simulink model "DecentralizedLFADRC"  (R2019b)
settings: Solver=ode4  StartTime=0.0  StopTime=480  FixedStep=1e-3  MaxStep=1e-4  RelTol=1e-3  EnableMultiTasking=on
values from neighbouring files (symbols this model uses):
  a_1 = 0.5    [system_parameters.m]
  a_10 = 0.125    [system_parameters.m]
  a_2 = 0.125    [system_parameters.m]
  a_3 = 0.125    [system_parameters.m]
  a_4 = 0.5    [system_parameters.m]
  a_5 = 0.1    [system_parameters.m]
  a_6 = 0.1    [system_parameters.m]
  a_7 = 0.1    [system_parameters.m]
  a_8 = 0.125    [system_parameters.m]
  a_9 = 0.5    [system_parameters.m]
  a_PV1 = 0.125    [system_parameters.m]
  a_PV2 = 0.2    [system_parameters.m]
  a_PV3 = 0.125    [system_parameters.m]
  a_WT1 = 0.125    [system_parameters.m]
  a_WT3 = 0.125    [system_parameters.m]
  B1 = (1/Req1)+D    [system_parameters.m]
  B2 = (1/Req2)+D    [system_parameters.m]
  B3 = (1/Req3)+D    [system_parameters.m]
  D = 2    [system_parameters.m]
  H_A1 = (H1*S1+H2*S2+H3*S3)/(S1+S2+S3)    (= 2.58715528865)    [system_parameters.m]
  H_A2 = (H4*S4+H5*S5+H6*S6+H7*S7)/(S4+S5+S6+S7)    (= 2.6419)    [system_parameters.m]
  H_A3 = (H8*S8+H9*S9+H10*S10)/(S8+S9+S10)    (= 2.49952427226)    [system_parameters.m]
  K1 = -K1    [design_LFADRC.m]
  K2 = -K2    [design_LFADRC.m]
  K3 = -K3    [design_LFADRC.m]
  kpc = 0.8    [system_parameters.m]
  R1 = 0.0548    [system_parameters.m]
  R4 = 0.06    [system_parameters.m]
  R9 = 0.0548    [system_parameters.m]
  Rp10 = 0.06    [system_parameters.m]
  Rp2 = 0.06    [system_parameters.m]
  Rp3 = 0.06    [system_parameters.m]
  Rp5 = 0.0548    [system_parameters.m]
  Rp6 = 0.06    [system_parameters.m]
  Rp7 = 0.06    [system_parameters.m]
  Rp8 = 0.06    [system_parameters.m]
  RPV1 = 0.05    [system_parameters.m]
  RPV2 = 0.05    [system_parameters.m]
  RPV3 = 0.05    [system_parameters.m]
  RWT1 = 0.024    [system_parameters.m]
  RWT3 = 0.024    [system_parameters.m]
  T12 = 2.5    [system_parameters.m]
  T13 = 5.0    (= 5)    [system_parameters.m]
  T23 = 3.8    [system_parameters.m]
undefined symbols (not defined in the file or in its folder): A_obs_1, A_obs_2, A_obs_3, B_obs_1, B_obs_2, B_obs_3, C_obs_1, C_obs_2, C_obs_3, D_obs_1, D_obs_2, D_obs_3, X_hat_1, X_hat_2, X_hat_3, Xi_hat_1, Xi_hat_2, Xi_hat_3
libraries: cstblocks x94, simulink x40
(part 1 of 2)
settings Model: Creator=sergi  LastModifiedBy=sergio.dorado
settings DataIOCC: LimitDataPoints=on  SaveFormat=Array  ReturnWorkspaceOutputs=off
settings OptimizationCC: LifeSpan=inf
settings DebuggingCC: SFUnexpectedBacktrackingDiag=warning  SFNoUnconditionalDefaultTransitionDiag=warning  SFExecutionAtInitializationDiag=none  ArithmeticOperatorsInVariantConditions=warning
settings HardwareCC: ProdBitPerPointer=32  ProdBitPerSizeT=32  ProdBitPerPtrDiffT=32  ProdLargestAtomicFloat=None  ProdIntDivRoundTo=Undefined  ProdEndianess=Unspecified  ProdWordSize=32  ProdHWDeviceType=32-bit Generic
settings ModelReferenceCC: PropagateSignalLabelsOutOfModel=off
settings SFSimCC: SimUseLocalCustomCode=off  CustomCodeUndefinedFunction=UseInterfaceOnly
settings RTWCC: RTWUseLocalCustomCode=off
settings CodeAppCC: StateflowObjectComments=on
settings GRTTargetCC: TargetLangStandard=C89/C90 (ANSI)  GeneratePreprocessorConditionals=Disable all
settings ConfigComp: CovMetricSettings=dw  CovHtmlReporting=on  CovSaveCumulativeToWorkspaceVar=on  CovSaveSingleToWorkspaceVar=on  CovExternalEMLEnable=off

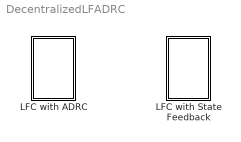
== system DecentralizedLFADRC ==
  LFC with State Feedback : Subsystem
  LFC with ADRC : Subsystem

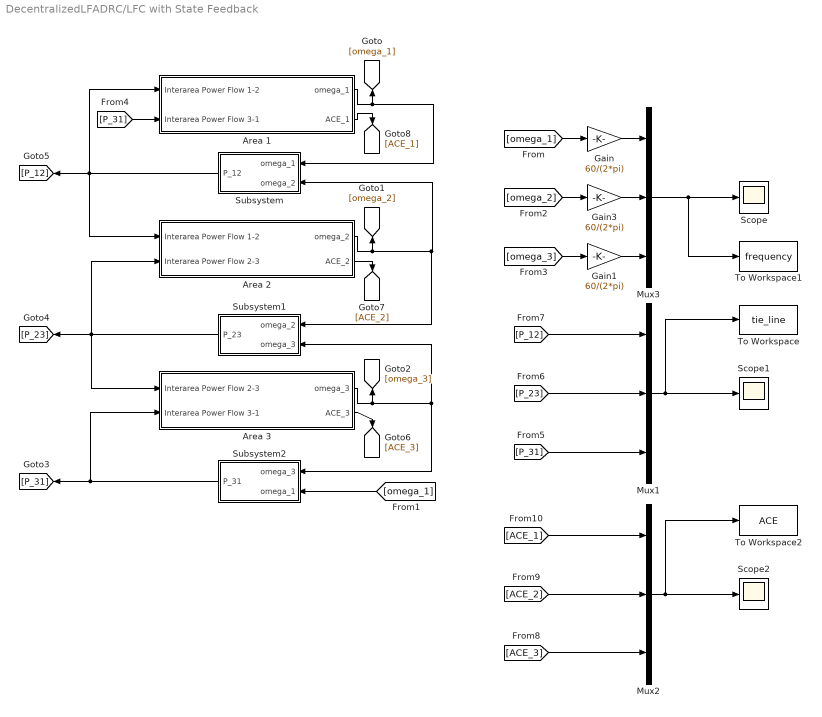
== system DecentralizedLFADRC/LFC with State Feedback ==
  Area 1 : Subsystem
  Area 2 : Subsystem
  Area 3 : Subsystem
  Gain : Gain  Gain=60/(2*pi)
  Gain1 : Gain  Gain=60/(2*pi)
  Gain3 : Gain  Gain=60/(2*pi)
  Mux1 : Mux  Inputs=3
  Mux2 : Mux  Inputs=3
  Mux3 : Mux  Inputs=3
  Scope : Scope
  Scope1 : Scope
  Scope2 : Scope
  Subsystem : Subsystem
  Subsystem1 : Subsystem
  Subsystem2 : Subsystem
  To Workspace : ToWorkspace  VariableName=tie_line  SaveFormat=Structure With Time  SampleTime=-1
  To Workspace1 : ToWorkspace  VariableName=frequency  SaveFormat=Structure With Time  SampleTime=-1
  To Workspace2 : ToWorkspace  VariableName=ACE  SaveFormat=Structure With Time  SampleTime=-1
  wires:
  Gain3/1 -> Mux3/2
  Area 3/1(omega_3) -> Subsystem2/1(omega_3), Subsystem1/2(omega_3), [omega_3]
  Mux3/1 -> To Workspace1/1, Scope/1
  [P_12] -> Mux1/1
  Mux1/1 -> To Workspace/1, Scope1/1
  [omega_1] -> Gain/1
  Area 2/1(omega_2) -> Subsystem1/1(omega_2), Subsystem/2(omega_2), [omega_2]
  Area 1/1(omega_1) -> Subsystem/1(omega_1), [omega_1]
  Gain/1 -> Mux3/1
  [P_31] -> Mux1/3
  Subsystem2/1(P_31) -> [P_31], Area 3/2(Interarea Power Flow 3-1)
  Subsystem/1(P_12) -> [P_12], Area 2/1(Interarea Power Flow 1-2), Area 1/1(Interarea Power Flow 1-2)
  [omega_2] -> Gain3/1
  [omega_1] -> Subsystem2/2(omega_1)
  [P_31] -> Area 1/2(Interarea Power Flow 3-1)
  [omega_3] -> Gain1/1
  Subsystem1/1(P_23) -> [P_23], Area 3/1(Interarea Power Flow 2-3), Area 2/2(Interarea Power Flow 2-3)
  Gain1/1 -> Mux3/3
  [P_23] -> Mux1/2
  [ACE_1] -> Mux2/1
  [ACE_2] -> Mux2/2
  [ACE_3] -> Mux2/3
  Mux2/1 -> Scope2/1, To Workspace2/1
  Area 3/2(ACE_3) -> [ACE_3]
  Area 2/2(ACE_2) -> [ACE_2]
  Area 1/2(ACE_1) -> [ACE_1]

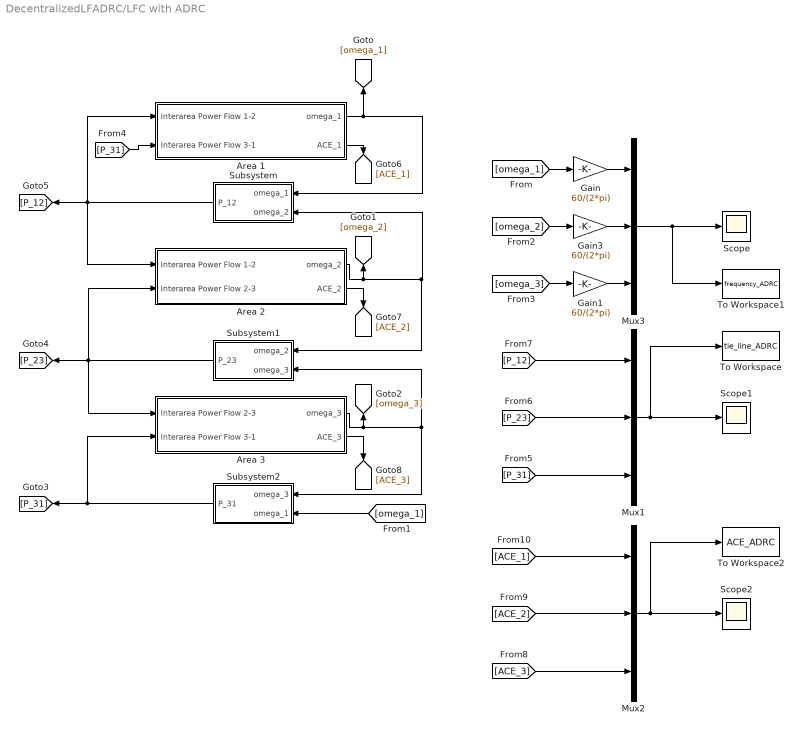
== system DecentralizedLFADRC/LFC with ADRC ==
  Area 1 : Subsystem
  Area 2 : Subsystem
  Area 3 : Subsystem
  Gain : Gain  Gain=60/(2*pi)
  Gain1 : Gain  Gain=60/(2*pi)
  Gain3 : Gain  Gain=60/(2*pi)
  Mux1 : Mux  Inputs=3
  Mux2 : Mux  Inputs=3
  Mux3 : Mux  Inputs=3
  Scope : Scope
  Scope1 : Scope
  Scope2 : Scope
  Subsystem : Subsystem
  Subsystem1 : Subsystem
  Subsystem2 : Subsystem
  To Workspace : ToWorkspace  VariableName=tie_line_ADRC  SaveFormat=Structure With Time  SampleTime=-1
  To Workspace1 : ToWorkspace  VariableName=frequency_ADRC  SaveFormat=Structure With Time  SampleTime=-1
  To Workspace2 : ToWorkspace  VariableName=ACE_ADRC  SaveFormat=Structure With Time  SampleTime=-1
  wires:
  [P_23] -> Mux1/2
  Gain1/1 -> Mux3/3
  Subsystem1/1(P_23) -> Area 2/2(Interarea Power Flow 2-3), Area 3/1(Interarea Power Flow 2-3), [P_23]
  [omega_3] -> Gain1/1
  [P_31] -> Area 1/2(Interarea Power Flow 3-1)
  [omega_1] -> Subsystem2/2(omega_1)
  [omega_2] -> Gain3/1
  Subsystem/1(P_12) -> Area 1/1(Interarea Power Flow 1-2), Area 2/1(Interarea Power Flow 1-2), [P_12]
  Subsystem2/1(P_31) -> Area 3/2(Interarea Power Flow 3-1), [P_31]
  [P_31] -> Mux1/3
  Gain/1 -> Mux3/1
  Area 1/1(omega_1) -> Subsystem/1(omega_1), [omega_1]
  Area 2/1(omega_2) -> [omega_2], Subsystem/2(omega_2), Subsystem1/1(omega_2)
  [omega_1] -> Gain/1
  Mux1/1 -> Scope1/1, To Workspace/1
  [P_12] -> Mux1/1
  Mux3/1 -> Scope/1, To Workspace1/1
  Area 3/1(omega_3) -> [omega_3], Subsystem1/2(omega_3), Subsystem2/1(omega_3)
  Gain3/1 -> Mux3/2
  [ACE_3] -> Mux2/3
  Mux2/1 -> Scope2/1, To Workspace2/1
  [ACE_1] -> Mux2/1
  [ACE_2] -> Mux2/2
  Area 1/2(ACE_1) -> [ACE_1]
  Area 2/2(ACE_2) -> [ACE_2]
  Area 3/2(ACE_3) -> [ACE_3]

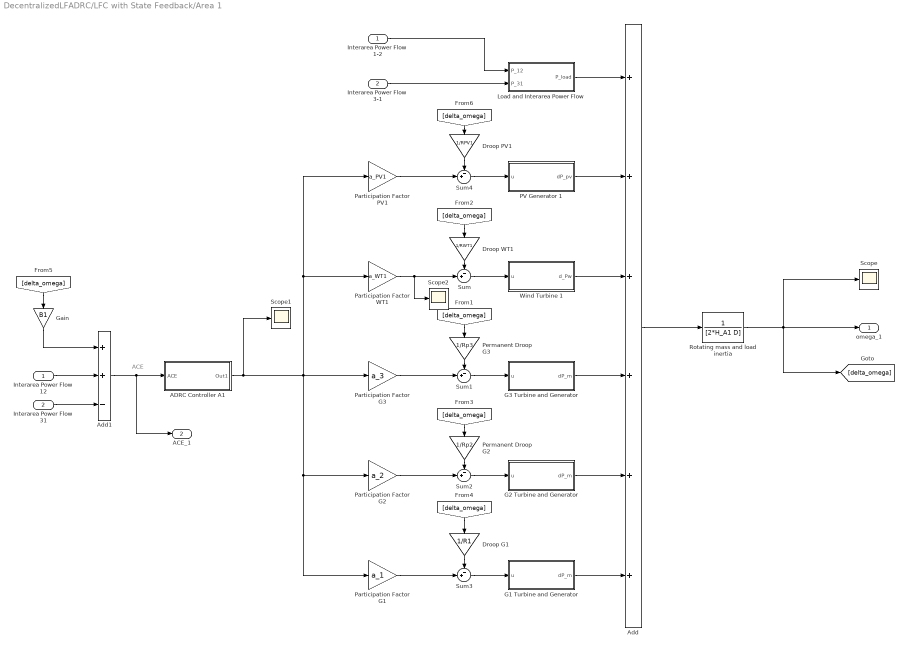
== system DecentralizedLFADRC/LFC with State Feedback/Area 1 ==
  note: ACE
  Interarea Power Flow 1-2 : Inport
  Interarea Power Flow 3-1 : Inport  Port=2
  ADRC Controller A1 : Subsystem
  Add : Sum  Inputs=6
  Add1 : Sum  Inputs=++-
  Droop G1 : Gain  Gain=1/R1
  Droop PV1 : Gain  Gain=1/RPV1
  Droop WT1 : Gain  Gain=1/RWT1
  G1 Turbine and Generator : Subsystem
  G2 Turbine and Generator : Subsystem
  G3 Turbine and Generator : Subsystem
  Gain : Gain  Gain=B1
  Interarea Power Flow 12 : InportShadow
  Interarea Power Flow 31 : InportShadow  Port=2
  Load and Interarea Power Flow : Subsystem
  "PV Generator 1 " : Subsystem
  Participation Factor G1 : Gain  Gain=a_1
  Participation Factor G2 : Gain  Gain=a_2
  Participation Factor G3 : Gain  Gain=a_3
  Participation Factor PV1 : Gain  Gain=a_PV1
  Participation Factor WT1 : Gain  Gain=a_WT1
  Permanent Droop G2 : Gain  Gain=1/Rp2
  Permanent Droop G3 : Gain  Gain=1/Rp3
  Rotating mass and load inertia : TransferFcn  Denominator=[2*H_A1 D]
  Scope : Scope
  Scope1 : Scope
  Scope2 : Scope
  Sum{,1..4} (5 alike) : Sum  Inputs=-+|
  Wind Turbine 1 : Subsystem
  omega_1 : Outport  VectorParamsAs1DForOutWhenUnconnected=off
  ACE_1 : Outport  Port=2  VectorParamsAs1DForOutWhenUnconnected=off
  wires:
  Rotating mass and load inertia/1 -> omega_1/1, Scope/1, [delta_omega]
  Add/1 -> Rotating mass and load inertia/1
  Sum/1 -> Wind Turbine 1/1(u)
  Sum1/1 -> G3 Turbine and Generator/1(u)
  Sum2/1 -> G2 Turbine and Generator/1(u)
  Droop G1/1 -> Sum3/1
  [delta_omega] -> Droop G1/1
  Participation Factor WT1/1 -> Scope2/1, Sum/2
  Participation Factor G3/1 -> Sum1/2
  Participation Factor G2/1 -> Sum2/2
  Participation Factor G1/1 -> Sum3/2
  Permanent Droop G2/1 -> Sum2/1
  [delta_omega] -> Permanent Droop G2/1
  Permanent Droop G3/1 -> Sum1/1
  [delta_omega] -> Permanent Droop G3/1
  Droop WT1/1 -> Sum/1
  [delta_omega] -> Droop WT1/1
  Interarea Power Flow 1-2/1 -> Load and Interarea Power Flow/1(P_12)
  Interarea Power Flow 3-1/1 -> Load and Interarea Power Flow/2(P_31)
  Sum3/1 -> G1 Turbine and Generator/1(u)
  G1 Turbine and Generator/1(dP_m) -> Add/6
  G2 Turbine and Generator/1(dP_m) -> Add/5
  G3 Turbine and Generator/1(dP_m) -> Add/4
  Wind Turbine 1/1(d_Pw) -> Add/3
  [delta_omega] -> Droop PV1/1
  Droop PV1/1 -> Sum4/1
  Participation Factor PV1/1 -> Sum4/2
  Sum4/1 -> "PV Generator 1 "/1(u)
  "PV Generator 1 "/1(dP_pv) -> Add/2
  Load and Interarea Power Flow/1(P_load) -> Add/1
  Add1/1 -> ACE_1/1, ADRC Controller A1/1(ACE)
  [delta_omega] -> Gain/1
  Gain/1 -> Add1/1
  Interarea Power Flow 31/1 -> Add1/3
  Interarea Power Flow 12/1 -> Add1/2
  ADRC Controller A1/1(Out1) -> Participation Factor WT1/1, Participation Factor PV1/1, Participation Factor G3/1, Participation Factor G1/1, Participation Factor G2/1, Scope1/1

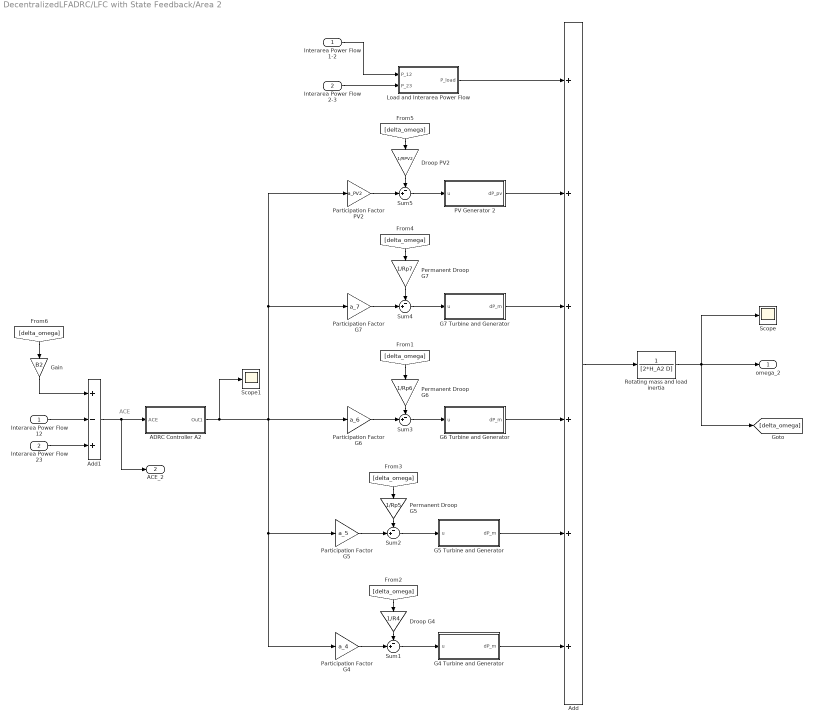
== system DecentralizedLFADRC/LFC with State Feedback/Area 2 ==
  note: ACE
  Interarea Power Flow 1-2 : Inport
  Interarea Power Flow 2-3 : Inport  Port=2
  ADRC Controller A2 : Subsystem
  Add : Sum  Inputs=6
  Add1 : Sum  Inputs=+-+
  Droop G4 : Gain  Gain=1/R4
  Droop PV2 : Gain  Gain=1/RPV2
  G4 Turbine and Generator : Subsystem
  G5 Turbine and Generator : Subsystem
  G6 Turbine and Generator : Subsystem
  G7 Turbine and Generator : Subsystem
  Gain : Gain  Gain=B2
  Interarea Power Flow 12 : InportShadow
  Interarea Power Flow 23 : InportShadow  Port=2
  Load and Interarea Power Flow : Subsystem
  "PV Generator 2 " : Subsystem
  Participation Factor G4 : Gain  Gain=a_4
  Participation Factor G5 : Gain  Gain=a_5
  Participation Factor G6 : Gain  Gain=a_6
  Participation Factor G7 : Gain  Gain=a_7
  Participation Factor PV2 : Gain  Gain=a_PV2
  Permanent Droop G5 : Gain  Gain=1/Rp5
  Permanent Droop G6 : Gain  Gain=1/Rp6
  Permanent Droop G7 : Gain  Gain=1/Rp7
  Rotating mass and load inertia : TransferFcn  Denominator=[2*H_A2 D]
  Scope : Scope
  Scope1 : Scope
  Sum{1..5} (5 alike) : Sum  Inputs=-+|
  omega_2 : Outport  VectorParamsAs1DForOutWhenUnconnected=off
  ACE_2 : Outport  Port=2  VectorParamsAs1DForOutWhenUnconnected=off
  wires:
  Add/1 -> Rotating mass and load inertia/1
  Rotating mass and load inertia/1 -> omega_2/1, Scope/1, [delta_omega]
  Sum4/1 -> G7 Turbine and Generator/1(u)
  Droop G4/1 -> Sum1/1
  [delta_omega] -> Droop G4/1
  Sum1/1 -> G4 Turbine and Generator/1(u)
  Participation Factor G4/1 -> Sum1/2
  Permanent Droop G5/1 -> Sum2/1
  [delta_omega] -> Permanent Droop G5/1
  Participation Factor G5/1 -> Sum2/2
  Sum2/1 -> G5 Turbine and Generator/1(u)
  Sum3/1 -> G6 Turbine and Generator/1(u)
  Permanent Droop G6/1 -> Sum3/1
  Participation Factor G6/1 -> Sum3/2
  [delta_omega] -> Permanent Droop G6/1
  [delta_omega] -> Permanent Droop G7/1
  Permanent Droop G7/1 -> Sum4/1
  Participation Factor G7/1 -> Sum4/2
  Sum5/1 -> "PV Generator 2 "/1(u)
  Participation Factor PV2/1 -> Sum5/2
  [delta_omega] -> Droop PV2/1
  Droop PV2/1 -> Sum5/1
  Load and Interarea Power Flow/1(P_load) -> Add/1
  ADRC Controller A2/1(Out1) -> Scope1/1, Participation Factor G4/1, Participation Factor G5/1, Participation Factor G6/1, Participation Factor PV2/1, Participation Factor G7/1
  Interarea Power Flow 2-3/1 -> Load and Interarea Power Flow/2(P_23)
  Interarea Power Flow 1-2/1 -> Load and Interarea Power Flow/1(P_12)
  G4 Turbine and Generator/1(dP_m) -> Add/6
  "PV Generator 2 "/1(dP_pv) -> Add/2
  Interarea Power Flow 23/1 -> Add1/3
  Gain/1 -> Add1/1
  Add1/1 -> ACE_2/1, ADRC Controller A2/1(ACE)
  Interarea Power Flow 12/1 -> Add1/2
  [delta_omega] -> Gain/1
  G7 Turbine and Generator/1(dP_m) -> Add/3
  G6 Turbine and Generator/1(dP_m) -> Add/4
  G5 Turbine and Generator/1(dP_m) -> Add/5

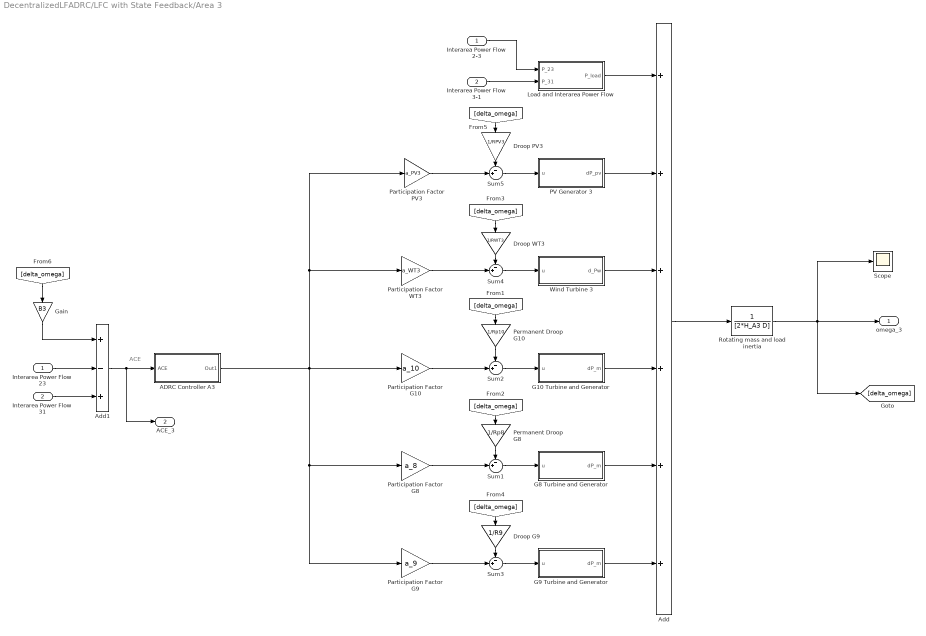
== system DecentralizedLFADRC/LFC with State Feedback/Area 3 ==
  note: ACE
  Interarea Power Flow 2-3 : Inport
  Interarea Power Flow 3-1 : Inport  Port=2
  ADRC Controller A3 : Subsystem
  Add : Sum  Inputs=6
  Add1 : Sum  Inputs=+-+
  Droop G9 : Gain  Gain=1/R9
  Droop PV3 : Gain  Gain=1/RPV3
  Droop WT3 : Gain  Gain=1/RWT3
  G10 Turbine and Generator : Subsystem
  G8 Turbine and Generator : Subsystem
  G9 Turbine and Generator : Subsystem
  Gain : Gain  Gain=B3
  Interarea Power Flow 23 : InportShadow
  Interarea Power Flow 31 : InportShadow  Port=2
  Load and Interarea Power Flow : Subsystem
  "PV Generator 3 " : Subsystem
  Participation Factor G10 : Gain  Gain=a_10
  Participation Factor G8 : Gain  Gain=a_8
  Participation Factor G9 : Gain  Gain=a_9
  Participation Factor PV3 : Gain  Gain=a_PV3
  Participation Factor WT3 : Gain  Gain=a_WT3
  Permanent Droop G10 : Gain  Gain=1/Rp10
  Permanent Droop G8 : Gain  Gain=1/Rp8
  Rotating mass and load inertia : TransferFcn  Denominator=[2*H_A3 D]
  Scope : Scope
  Sum{1..5} (5 alike) : Sum  Inputs=-+|
  Wind Turbine 3 : Subsystem
  omega_3 : Outport  VectorParamsAs1DForOutWhenUnconnected=off
  ACE_3 : Outport  Port=2  VectorParamsAs1DForOutWhenUnconnected=off
  wires:
  Rotating mass and load inertia/1 -> [delta_omega], omega_3/1, Scope/1
  Droop G9/1 -> Sum3/1
  [delta_omega] -> Droop G9/1
  Sum3/1 -> G9 Turbine and Generator/1(u)
  Participation Factor G9/1 -> Sum3/2
  Permanent Droop G8/1 -> Sum1/1
  [delta_omega] -> Permanent Droop G8/1
  Sum1/1 -> G8 Turbine and Generator/1(u)
  Participation Factor G8/1 -> Sum1/2
  Load and Interarea Power Flow/1(P_load) -> Add/1
  Permanent Droop G10/1 -> Sum2/1
  [delta_omega] -> Permanent Droop G10/1
  Sum2/1 -> G10 Turbine and Generator/1(u)
  Participation Factor G10/1 -> Sum2/2
  Droop WT3/1 -> Sum4/1
  [delta_omega] -> Droop WT3/1
  Sum4/1 -> Wind Turbine 3/1(u)
  Participation Factor WT3/1 -> Sum4/2
  Interarea Power Flow 2-3/1 -> Load and Interarea Power Flow/1(P_23)
  Interarea Power Flow 3-1/1 -> Load and Interarea Power Flow/2(P_31)
  Add/1 -> Rotating mass and load inertia/1
  G9 Turbine and Generator/1(dP_m) -> Add/6
  G8 Turbine and Generator/1(dP_m) -> Add/5
  G10 Turbine and Generator/1(dP_m) -> Add/4
  Wind Turbine 3/1(d_Pw) -> Add/3
  ADRC Controller A3/1(Out1) -> Participation Factor G9/1, Participation Factor G8/1, Participation Factor PV3/1, Participation Factor WT3/1, Participation Factor G10/1
  Droop PV3/1 -> Sum5/1
  [delta_omega] -> Droop PV3/1
  "PV Generator 3 "/1(dP_pv) -> Add/2
  Sum5/1 -> "PV Generator 3 "/1(u)
  Participation Factor PV3/1 -> Sum5/2
  Add1/1 -> ACE_3/1, ADRC Controller A3/1(ACE)
  [delta_omega] -> Gain/1
  Gain/1 -> Add1/1
  Interarea Power Flow 31/1 -> Add1/3
  Interarea Power Flow 23/1 -> Add1/2

== system DecentralizedLFADRC/LFC with State Feedback/Subsystem ==
  omega_1 : Inport
  omega_2 : Inport  Port=2
  Add : Sum  Inputs=+-
  Gain : Gain  Gain=T12
  Integrator2 : Integrator
  P_12 : Outport  VectorParamsAs1DForOutWhenUnconnected=off
  wires:
  Add/1 -> Integrator2/1
  omega_1/1 -> Add/1
  omega_2/1 -> Add/2
  Gain/1 -> P_12/1
  Integrator2/1 -> Gain/1

== system DecentralizedLFADRC/LFC with State Feedback/Subsystem1 ==
  omega_2 : Inport
  omega_3 : Inport  Port=2
  Add : Sum  Inputs=+-
  Gain : Gain  Gain=T23
  Integrator2 : Integrator
  P_23 : Outport  VectorParamsAs1DForOutWhenUnconnected=off
  wires:
  Integrator2/1 -> Gain/1
  Gain/1 -> P_23/1
  omega_3/1 -> Add/2
  omega_2/1 -> Add/1
  Add/1 -> Integrator2/1

== system DecentralizedLFADRC/LFC with State Feedback/Subsystem2 ==
  omega_3 : Inport
  omega_1 : Inport  Port=2
  Add : Sum  Inputs=+-
  Gain : Gain  Gain=T13
  Integrator2 : Integrator
  P_31 : Outport  VectorParamsAs1DForOutWhenUnconnected=off
  wires:
  Add/1 -> Integrator2/1
  omega_3/1 -> Add/1
  omega_1/1 -> Add/2
  Gain/1 -> P_31/1
  Integrator2/1 -> Gain/1

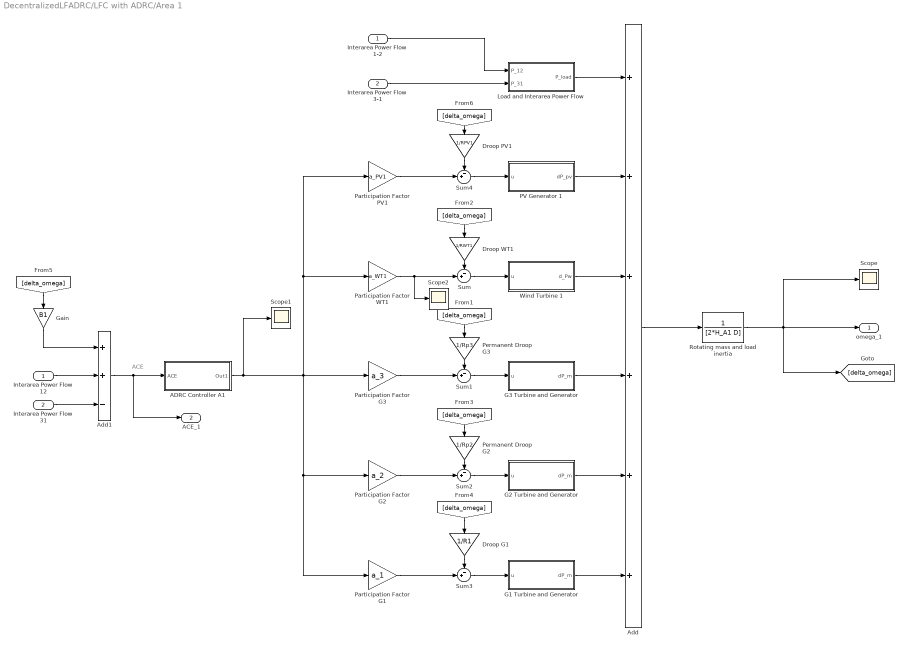
== system DecentralizedLFADRC/LFC with ADRC/Area 1 ==
  note: ACE
  Interarea Power Flow 1-2 : Inport
  Interarea Power Flow 3-1 : Inport  Port=2
  ADRC Controller A1 : Subsystem
  Add : Sum  Inputs=6
  Add1 : Sum  Inputs=++-
  Droop G1 : Gain  Gain=1/R1
  Droop PV1 : Gain  Gain=1/RPV1
  Droop WT1 : Gain  Gain=1/RWT1
  G1 Turbine and Generator : Subsystem
  G2 Turbine and Generator : Subsystem
  G3 Turbine and Generator : Subsystem
  Gain : Gain  Gain=B1
  Interarea Power Flow 12 : InportShadow
  Interarea Power Flow 31 : InportShadow  Port=2
  Load and Interarea Power Flow : Subsystem
  "PV Generator 1 " : Subsystem
  Participation Factor G1 : Gain  Gain=a_1
  Participation Factor G2 : Gain  Gain=a_2
  Participation Factor G3 : Gain  Gain=a_3
  Participation Factor PV1 : Gain  Gain=a_PV1
  Participation Factor WT1 : Gain  Gain=a_WT1
  Permanent Droop G2 : Gain  Gain=1/Rp2
  Permanent Droop G3 : Gain  Gain=1/Rp3
  Rotating mass and load inertia : TransferFcn  Denominator=[2*H_A1 D]
  Scope : Scope
  Scope1 : Scope
  Scope2 : Scope
  Sum{,1..4} (5 alike) : Sum  Inputs=-+|
  Wind Turbine 1 : Subsystem
  omega_1 : Outport  VectorParamsAs1DForOutWhenUnconnected=off
  ACE_1 : Outport  Port=2  VectorParamsAs1DForOutWhenUnconnected=off
  wires:
  ADRC Controller A1/1(Out1) -> Scope1/1, Participation Factor G2/1, Participation Factor G1/1, Participation Factor G3/1, Participation Factor PV1/1, Participation Factor WT1/1
  Interarea Power Flow 12/1 -> Add1/2
  Interarea Power Flow 31/1 -> Add1/3
  Gain/1 -> Add1/1
  [delta_omega] -> Gain/1
  Add1/1 -> ACE_1/1, ADRC Controller A1/1(ACE)
  Load and Interarea Power Flow/1(P_load) -> Add/1
  "PV Generator 1 "/1(dP_pv) -> Add/2
  Sum4/1 -> "PV Generator 1 "/1(u)
  Participation Factor PV1/1 -> Sum4/2
  Droop PV1/1 -> Sum4/1
  [delta_omega] -> Droop PV1/1
  Wind Turbine 1/1(d_Pw) -> Add/3
  G3 Turbine and Generator/1(dP_m) -> Add/4
  G2 Turbine and Generator/1(dP_m) -> Add/5
  G1 Turbine and Generator/1(dP_m) -> Add/6
  Sum3/1 -> G1 Turbine and Generator/1(u)
  Interarea Power Flow 3-1/1 -> Load and Interarea Power Flow/2(P_31)
  Interarea Power Flow 1-2/1 -> Load and Interarea Power Flow/1(P_12)
  [delta_omega] -> Droop WT1/1
  Droop WT1/1 -> Sum/1
  [delta_omega] -> Permanent Droop G3/1
  Permanent Droop G3/1 -> Sum1/1
  [delta_omega] -> Permanent Droop G2/1
  Permanent Droop G2/1 -> Sum2/1
  Participation Factor G1/1 -> Sum3/2
  Participation Factor G2/1 -> Sum2/2
  Participation Factor G3/1 -> Sum1/2
  Participation Factor WT1/1 -> Sum/2, Scope2/1
  [delta_omega] -> Droop G1/1
  Droop G1/1 -> Sum3/1
  Sum2/1 -> G2 Turbine and Generator/1(u)
  Sum1/1 -> G3 Turbine and Generator/1(u)
  Sum/1 -> Wind Turbine 1/1(u)
  Add/1 -> Rotating mass and load inertia/1
  Rotating mass and load inertia/1 -> [delta_omega], Scope/1, omega_1/1

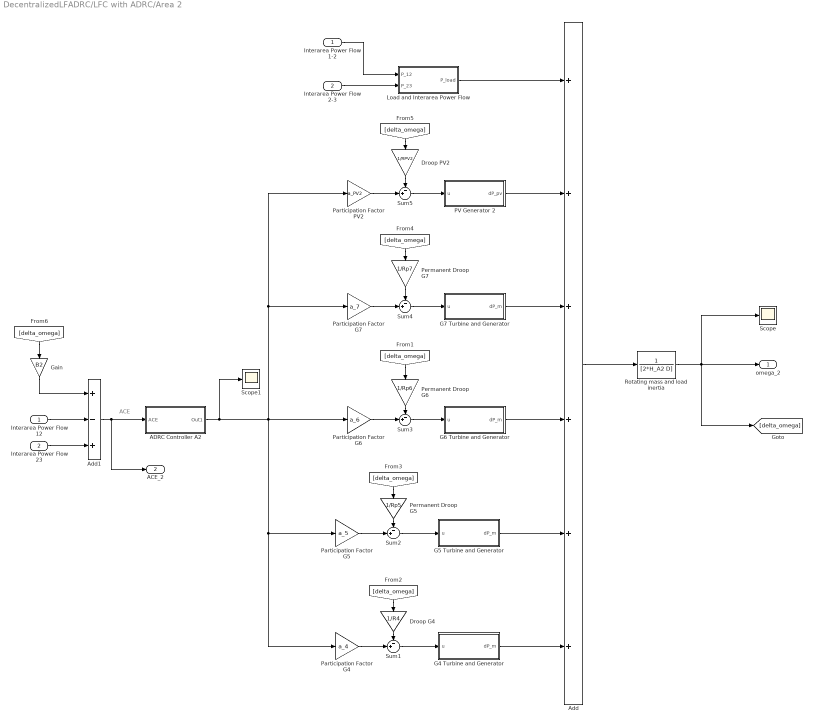
== system DecentralizedLFADRC/LFC with ADRC/Area 2 ==
  note: ACE
  Interarea Power Flow 1-2 : Inport
  Interarea Power Flow 2-3 : Inport  Port=2
  ADRC Controller A2 : Subsystem
  Add : Sum  Inputs=6
  Add1 : Sum  Inputs=+-+
  Droop G4 : Gain  Gain=1/R4
  Droop PV2 : Gain  Gain=1/RPV2
  G4 Turbine and Generator : Subsystem
  G5 Turbine and Generator : Subsystem
  G6 Turbine and Generator : Subsystem
  G7 Turbine and Generator : Subsystem
  Gain : Gain  Gain=B2
  Interarea Power Flow 12 : InportShadow
  Interarea Power Flow 23 : InportShadow  Port=2
  Load and Interarea Power Flow : Subsystem
  "PV Generator 2 " : Subsystem
  Participation Factor G4 : Gain  Gain=a_4
  Participation Factor G5 : Gain  Gain=a_5
  Participation Factor G6 : Gain  Gain=a_6
  Participation Factor G7 : Gain  Gain=a_7
  Participation Factor PV2 : Gain  Gain=a_PV2
  Permanent Droop G5 : Gain  Gain=1/Rp5
  Permanent Droop G6 : Gain  Gain=1/Rp6
  Permanent Droop G7 : Gain  Gain=1/Rp7
  Rotating mass and load inertia : TransferFcn  Denominator=[2*H_A2 D]
  Scope : Scope
  Scope1 : Scope
  Sum{1..5} (5 alike) : Sum  Inputs=-+|
  omega_2 : Outport  VectorParamsAs1DForOutWhenUnconnected=off
  ACE_2 : Outport  Port=2  VectorParamsAs1DForOutWhenUnconnected=off
  wires:
  G5 Turbine and Generator/1(dP_m) -> Add/5
  G6 Turbine and Generator/1(dP_m) -> Add/4
  G7 Turbine and Generator/1(dP_m) -> Add/3
  [delta_omega] -> Gain/1
  Interarea Power Flow 12/1 -> Add1/2
  Add1/1 -> ACE_2/1, ADRC Controller A2/1(ACE)
  Gain/1 -> Add1/1
  Interarea Power Flow 23/1 -> Add1/3
  "PV Generator 2 "/1(dP_pv) -> Add/2
  G4 Turbine and Generator/1(dP_m) -> Add/6
  Interarea Power Flow 1-2/1 -> Load and Interarea Power Flow/1(P_12)
  Interarea Power Flow 2-3/1 -> Load and Interarea Power Flow/2(P_23)
  ADRC Controller A2/1(Out1) -> Participation Factor G7/1, Participation Factor PV2/1, Participation Factor G6/1, Participation Factor G5/1, Participation Factor G4/1, Scope1/1
  Load and Interarea Power Flow/1(P_load) -> Add/1
  Droop PV2/1 -> Sum5/1
  [delta_omega] -> Droop PV2/1
  Participation Factor PV2/1 -> Sum5/2
  Sum5/1 -> "PV Generator 2 "/1(u)
  Participation Factor G7/1 -> Sum4/2
  Permanent Droop G7/1 -> Sum4/1
  [delta_omega] -> Permanent Droop G7/1
  [delta_omega] -> Permanent Droop G6/1
  Participation Factor G6/1 -> Sum3/2
  Permanent Droop G6/1 -> Sum3/1
  Sum3/1 -> G6 Turbine and Generator/1(u)
  Sum2/1 -> G5 Turbine and Generator/1(u)
  Participation Factor G5/1 -> Sum2/2
  [delta_omega] -> Permanent Droop G5/1
  Permanent Droop G5/1 -> Sum2/1
  Participation Factor G4/1 -> Sum1/2
  Sum1/1 -> G4 Turbine and Generator/1(u)
  [delta_omega] -> Droop G4/1
  Droop G4/1 -> Sum1/1
  Sum4/1 -> G7 Turbine and Generator/1(u)
  Rotating mass and load inertia/1 -> [delta_omega], Scope/1, omega_2/1
  Add/1 -> Rotating mass and load inertia/1

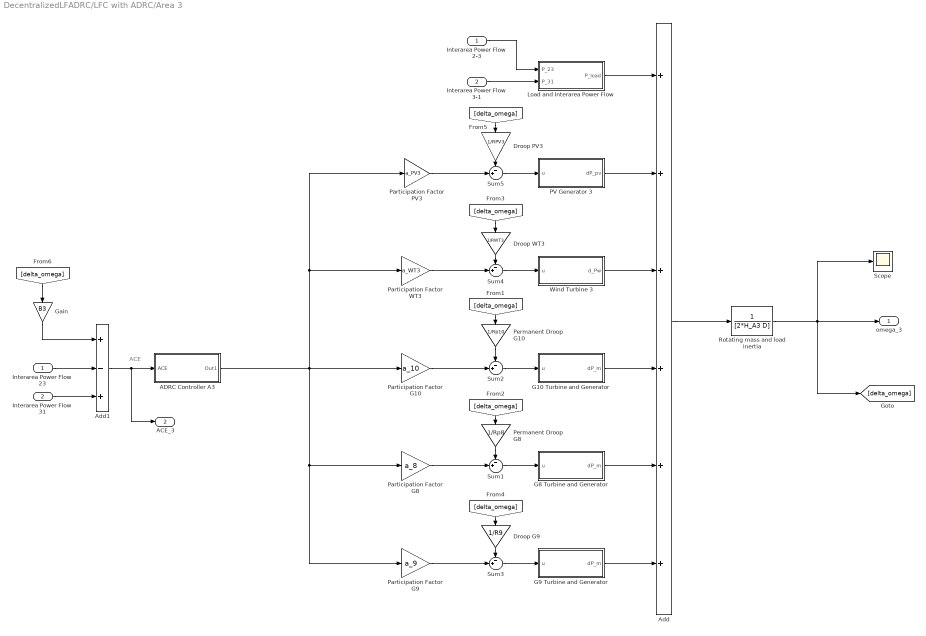
== system DecentralizedLFADRC/LFC with ADRC/Area 3 ==
  note: ACE
  Interarea Power Flow 2-3 : Inport
  Interarea Power Flow 3-1 : Inport  Port=2
  ADRC Controller A3 : Subsystem
  Add : Sum  Inputs=6
  Add1 : Sum  Inputs=+-+
  Droop G9 : Gain  Gain=1/R9
  Droop PV3 : Gain  Gain=1/RPV3
  Droop WT3 : Gain  Gain=1/RWT3
  G10 Turbine and Generator : Subsystem
  G8 Turbine and Generator : Subsystem
  G9 Turbine and Generator : Subsystem
  Gain : Gain  Gain=B3
  Interarea Power Flow 23 : InportShadow
  Interarea Power Flow 31 : InportShadow  Port=2
  Load and Interarea Power Flow : Subsystem
  "PV Generator 3 " : Subsystem
  Participation Factor G10 : Gain  Gain=a_10
  Participation Factor G8 : Gain  Gain=a_8
  Participation Factor G9 : Gain  Gain=a_9
  Participation Factor PV3 : Gain  Gain=a_PV3
  Participation Factor WT3 : Gain  Gain=a_WT3
  Permanent Droop G10 : Gain  Gain=1/Rp10
  Permanent Droop G8 : Gain  Gain=1/Rp8
  Rotating mass and load inertia : TransferFcn  Denominator=[2*H_A3 D]
  Scope : Scope
  Sum{1..5} (5 alike) : Sum  Inputs=-+|
  Wind Turbine 3 : Subsystem
  omega_3 : Outport  VectorParamsAs1DForOutWhenUnconnected=off
  ACE_3 : Outport  Port=2  VectorParamsAs1DForOutWhenUnconnected=off
  wires:
  Interarea Power Flow 23/1 -> Add1/2
  Interarea Power Flow 31/1 -> Add1/3
  Gain/1 -> Add1/1
  [delta_omega] -> Gain/1
  Add1/1 -> ACE_3/1, ADRC Controller A3/1(ACE)
  Participation Factor PV3/1 -> Sum5/2
  Sum5/1 -> "PV Generator 3 "/1(u)
  "PV Generator 3 "/1(dP_pv) -> Add/2
  [delta_omega] -> Droop PV3/1
  Droop PV3/1 -> Sum5/1
  ADRC Controller A3/1(Out1) -> Participation Factor G10/1, Participation Factor WT3/1, Participation Factor PV3/1, Participation Factor G8/1, Participation Factor G9/1
  Wind Turbine 3/1(d_Pw) -> Add/3
  G10 Turbine and Generator/1(dP_m) -> Add/4
  G8 Turbine and Generator/1(dP_m) -> Add/5
  G9 Turbine and Generator/1(dP_m) -> Add/6
  Add/1 -> Rotating mass and load inertia/1
  Interarea Power Flow 3-1/1 -> Load and Interarea Power Flow/2(P_31)
  Interarea Power Flow 2-3/1 -> Load and Interarea Power Flow/1(P_23)
  Participation Factor WT3/1 -> Sum4/2
  Sum4/1 -> Wind Turbine 3/1(u)
  [delta_omega] -> Droop WT3/1
  Droop WT3/1 -> Sum4/1
  Participation Factor G10/1 -> Sum2/2
  Sum2/1 -> G10 Turbine and Generator/1(u)
  [delta_omega] -> Permanent Droop G10/1
  Permanent Droop G10/1 -> Sum2/1
  Load and Interarea Power Flow/1(P_load) -> Add/1
  Participation Factor G8/1 -> Sum1/2
  Sum1/1 -> G8 Turbine and Generator/1(u)
  [delta_omega] -> Permanent Droop G8/1
  Permanent Droop G8/1 -> Sum1/1
  Participation Factor G9/1 -> Sum3/2
  Sum3/1 -> G9 Turbine and Generator/1(u)
  [delta_omega] -> Droop G9/1
  Droop G9/1 -> Sum3/1
  Rotating mass and load inertia/1 -> Scope/1, omega_3/1, [delta_omega]

== system DecentralizedLFADRC/LFC with ADRC/Subsystem ==
  omega_1 : Inport
  omega_2 : Inport  Port=2
  Add : Sum  Inputs=+-
  Gain : Gain  Gain=T12
  Integrator2 : Integrator
  P_12 : Outport  VectorParamsAs1DForOutWhenUnconnected=off
  wires:
  Integrator2/1 -> Gain/1
  Gain/1 -> P_12/1
  omega_2/1 -> Add/2
  omega_1/1 -> Add/1
  Add/1 -> Integrator2/1

== system DecentralizedLFADRC/LFC with ADRC/Subsystem1 ==
  omega_2 : Inport
  omega_3 : Inport  Port=2
  Add : Sum  Inputs=+-
  Gain : Gain  Gain=T23
  Integrator2 : Integrator
  P_23 : Outport  VectorParamsAs1DForOutWhenUnconnected=off
  wires:
  Add/1 -> Integrator2/1
  omega_2/1 -> Add/1
  omega_3/1 -> Add/2
  Gain/1 -> P_23/1
  Integrator2/1 -> Gain/1

== system DecentralizedLFADRC/LFC with ADRC/Subsystem2 ==
  omega_3 : Inport
  omega_1 : Inport  Port=2
  Add : Sum  Inputs=+-
  Gain : Gain  Gain=T13
  Integrator2 : Integrator
  P_31 : Outport  VectorParamsAs1DForOutWhenUnconnected=off
  wires:
  Integrator2/1 -> Gain/1
  Gain/1 -> P_31/1
  omega_1/1 -> Add/2
  omega_3/1 -> Add/1
  Add/1 -> Integrator2/1

== system DecentralizedLFADRC/LFC with State Feedback/Area 1/ADRC Controller A1 ==
  ACE : Inport
  Add : Sum  Inputs=-+
  Estimated State : Gain  Gain=X_hat_1  Multiplication=Matrix(K*u) (u vector)
  Estimated disturbance : Gain  Commented=on  Gain=Xi_hat_1  Multiplication=Matrix(K*u) (u vector)
  Mux : Mux  Inputs=2
  State Feedback Gain : Gain  Gain=K1  Multiplication=Matrix(K*u)
  State-Space : StateSpace  A=A_obs_1  B=B_obs_1  C=C_obs_1  D=D_obs_1  InitialCondition=0
  Out1 : Outport  VectorParamsAs1DForOutWhenUnconnected=off
  wires:
  State-Space/1 -> Estimated disturbance/1, Estimated State/1
  Estimated disturbance/1 -> Add/1
  Estimated State/1 -> State Feedback Gain/1
  State Feedback Gain/1 -> Add/2
  Add/1 -> Out1/1, Mux/1
  ACE/1 -> Mux/2
  Mux/1 -> State-Space/1

== system DecentralizedLFADRC/LFC with State Feedback/Area 1/G1 Turbine and Generator ==
  u : Inport
  G1 Governor : cstblocks/LTI System  sys=Gg1  IC=[]
  G1 Turbine : cstblocks/LTI System  sys=Gt1  IC=[]
  dP_m : Outport  VectorParamsAs1DForOutWhenUnconnected=off
  wires:
  G1 Turbine/1 -> dP_m/1
  G1 Governor/1 -> G1 Turbine/1
  u/1 -> G1 Governor/1

== system DecentralizedLFADRC/LFC with State Feedback/Area 1/G2 Turbine and Generator ==
  u : Inport
  G2 Governor : cstblocks/LTI System  sys=Gg2  IC=[]
  G2 Transient Droop Compensation : cstblocks/LTI System  sys=Gdc2  IC=[]
  G2 Turbine : cstblocks/LTI System  sys=Gt2  IC=[]
  dP_m : Outport  VectorParamsAs1DForOutWhenUnconnected=off
  wires:
  G2 Governor/1 -> G2 Transient Droop Compensation/1
  G2 Turbine/1 -> dP_m/1
  G2 Transient Droop Compensation/1 -> G2 Turbine/1
  u/1 -> G2 Governor/1

== system DecentralizedLFADRC/LFC with State Feedback/Area 1/G3 Turbine and Generator ==
  u : Inport
  G3 Governor : cstblocks/LTI System  sys=Gg3  IC=[]
  G3 Transient Droop Compensation : cstblocks/LTI System  sys=Gdc3  IC=[]
  G3 Turbine : cstblocks/LTI System  sys=Gt3  IC=[]
  dP_m : Outport  VectorParamsAs1DForOutWhenUnconnected=off
  wires:
  G3 Turbine/1 -> dP_m/1
  G3 Governor/1 -> G3 Transient Droop Compensation/1
  G3 Transient Droop Compensation/1 -> G3 Turbine/1
  u/1 -> G3 Governor/1

== system DecentralizedLFADRC/LFC with State Feedback/Area 1/Load and Interarea Power Flow ==
  P_12 : Inport
  P_31 : Inport  Port=2
  Add : Sum  Inputs=-+
  Add1 : Sum  Inputs=+++
  Gain1 : Gain  Gain=-1
  LTI System : cstblocks/LTI System  sys=tf(10,conv([1 10],[1 10]))  IC=[]
  "Load Disturbance Area 1 " : Subsystem
  PV Negative Load Area 1 : Subsystem
  Random Number : RandomNumber  Mean=10  Variance=10  SampleTime=5
  Rate Transition : RateTransition
  Scope1 : Scope
  P_load : Outport  VectorParamsAs1DForOutWhenUnconnected=off
  wires:
  "Load Disturbance Area 1 "/1(P_load) -> Gain1/1
  Gain1/1 -> Add1/2
  PV Negative Load Area 1/1(P_pv) -> Add1/3, Scope1/1
  P_12/1 -> Add/1
  P_31/1 -> Add/2
  Add/1 -> Add1/1
  Add1/1 -> P_load/1
  LTI System/1 -> PV Negative Load Area 1/1(Irradiance)
  Random Number/1 -> Rate Transition/1
  Rate Transition/1 -> LTI System/1

== system DecentralizedLFADRC/LFC with State Feedback/Area 1/PV Generator 1  ==
  u : Inport
  PV Dynamics for LFC Participation : cstblocks/LTI System  sys=Gpv_LFC  IC=[]
  dP_pv : Outport  VectorParamsAs1DForOutWhenUnconnected=off
  wires:
  PV Dynamics for LFC Participation/1 -> dP_pv/1
  u/1 -> PV Dynamics for LFC Participation/1

== system DecentralizedLFADRC/LFC with State Feedback/Area 1/Wind Turbine 1 ==
  u : Inport
  Blade Characteristic : Gain  Gain=kpc
  First order lag : cstblocks/LTI System  sys=Gwl  IC=[]
  Pitch actuator : cstblocks/LTI System  sys=Gwp  IC=[]
  d_Pw : Outport  VectorParamsAs1DForOutWhenUnconnected=off
  wires:
  Pitch actuator/1 -> First order lag/1
  u/1 -> Pitch actuator/1
  First order lag/1 -> Blade Characteristic/1
  Blade Characteristic/1 -> d_Pw/1

== system DecentralizedLFADRC/LFC with State Feedback/Area 2/ADRC Controller A2 ==
  ACE : Inport
  Add : Sum  Inputs=-+
  Estimated State : Gain  Gain=X_hat_2  Multiplication=Matrix(K*u) (u vector)
  Estimated disturbance : Gain  Commented=on  Gain=Xi_hat_2  Multiplication=Matrix(K*u) (u vector)
  Extended-State Observer Controller A2 : StateSpace  A=A_obs_2  B=B_obs_2  C=C_obs_2  D=D_obs_2  InitialCondition=0
  Mux : Mux  Inputs=2
  State Feedback Gain : Gain  Gain=K2  Multiplication=Matrix(K*u)
  Out1 : Outport  VectorParamsAs1DForOutWhenUnconnected=off
  wires:
  Extended-State Observer Controller A2/1 -> Estimated disturbance/1, Estimated State/1
  Estimated disturbance/1 -> Add/1
  Estimated State/1 -> State Feedback Gain/1
  State Feedback Gain/1 -> Add/2
  Add/1 -> Out1/1, Mux/1
  ACE/1 -> Mux/2
  Mux/1 -> Extended-State Observer Controller A2/1

== system DecentralizedLFADRC/LFC with State Feedback/Area 2/G4 Turbine and Generator ==
  u : Inport
  G4 Governor : cstblocks/LTI System  sys=Gg4  IC=[]
  G4 Turbine : cstblocks/LTI System  sys=Gt4  IC=[]
  dP_m : Outport  VectorParamsAs1DForOutWhenUnconnected=off
  wires:
  G4 Turbine/1 -> dP_m/1
  G4 Governor/1 -> G4 Turbine/1
  u/1 -> G4 Governor/1

== system DecentralizedLFADRC/LFC with State Feedback/Area 2/G5 Turbine and Generator ==
  u : Inport
  G5 Governor : cstblocks/LTI System  sys=Gg5  IC=[]
  G5 Transient Droop Compensation : cstblocks/LTI System  sys=Gdc5  IC=[]
  G5 Turbine : cstblocks/LTI System  sys=Gt5  IC=[]
  dP_m : Outport  VectorParamsAs1DForOutWhenUnconnected=off
  wires:
  u/1 -> G5 Governor/1
  G5 Transient Droop Compensation/1 -> G5 Turbine/1
  G5 Turbine/1 -> dP_m/1
  G5 Governor/1 -> G5 Transient Droop Compensation/1

== system DecentralizedLFADRC/LFC with State Feedback/Area 2/G6 Turbine and Generator ==
  u : Inport
  G6 Governor : cstblocks/LTI System  sys=Gg6  IC=[]
  G6 Transient Droop Compensation : cstblocks/LTI System  sys=Gdc6  IC=[]
  G6 Turbine : cstblocks/LTI System  sys=Gt6  IC=[]
  dP_m : Outport  VectorParamsAs1DForOutWhenUnconnected=off
  wires:
  u/1 -> G6 Governor/1
  G6 Transient Droop Compensation/1 -> G6 Turbine/1
  G6 Turbine/1 -> dP_m/1
  G6 Governor/1 -> G6 Transient Droop Compensation/1

== system DecentralizedLFADRC/LFC with State Feedback/Area 2/G7 Turbine and Generator ==
  u : Inport
  G7 Governor : cstblocks/LTI System  sys=Gg7  IC=[]
  G7 Transient Droop Compensation : cstblocks/LTI System  sys=Gdc7  IC=[]
  G7 Turbine : cstblocks/LTI System  sys=Gt7  IC=[]
  dP_m : Outport  VectorParamsAs1DForOutWhenUnconnected=off
  wires:
  G7 Governor/1 -> G7 Transient Droop Compensation/1
  G7 Turbine/1 -> dP_m/1
  G7 Transient Droop Compensation/1 -> G7 Turbine/1
  u/1 -> G7 Governor/1

== system DecentralizedLFADRC/LFC with State Feedback/Area 2/Load and Interarea Power Flow ==
  P_12 : Inport
  P_23 : Inport  Port=2
  Add : Sum  Inputs=+-
  Add1 : Sum  Inputs=+++
  Gain1 : Gain  Gain=-1
  LTI System : cstblocks/LTI System  sys=tf(10,conv([1 10],[1 10]))  IC=[]
  "Load Disturbance Area 2 " : Subsystem
  PV Negative Load Area 2 : Subsystem
  Random Number : RandomNumber  Mean=15  Variance=15  SampleTime=10
  Rate Transition : RateTransition
  Scope : Scope
  P_load : Outport  VectorParamsAs1DForOutWhenUnconnected=off
  wires:
  "Load Disturbance Area 2 "/1(P_load) -> Gain1/1
  Gain1/1 -> Add1/2
  PV Negative Load Area 2/1(P_pv) -> Add1/3
  P_12/1 -> Add/1
  P_23/1 -> Add/2
  Add/1 -> Add1/1
  Add1/1 -> P_load/1
  LTI System/1 -> Scope/1, PV Negative Load Area 2/1(Irradiance)
  Random Number/1 -> Rate Transition/1
  Rate Transition/1 -> LTI System/1

== system DecentralizedLFADRC/LFC with State Feedback/Area 2/PV Generator 2  ==
  u : Inport
  PV Dynamics for LFC Participation : cstblocks/LTI System  sys=Gpv_LFC  IC=[]
  dP_pv : Outport  VectorParamsAs1DForOutWhenUnconnected=off
  wires:
  PV Dynamics for LFC Participation/1 -> dP_pv/1
  u/1 -> PV Dynamics for LFC Participation/1

== system DecentralizedLFADRC/LFC with State Feedback/Area 3/ADRC Controller A3 ==
  ACE : Inport
  Add : Sum  Inputs=-+
  Estimated State : Gain  Gain=X_hat_3  Multiplication=Matrix(K*u) (u vector)
  Estimated disturbance : Gain  Commented=on  Gain=Xi_hat_3  Multiplication=Matrix(K*u) (u vector)
  Extended-State Observer Controller A3 : StateSpace  A=A_obs_3  B=B_obs_3  C=C_obs_3  D=D_obs_3  InitialCondition=0
  Mux : Mux  Inputs=2
  State Feedback Gain : Gain  Gain=K3  Multiplication=Matrix(K*u)
  Out1 : Outport  VectorParamsAs1DForOutWhenUnconnected=off
  wires:
  Extended-State Observer Controller A3/1 -> Estimated disturbance/1, Estimated State/1
  Estimated disturbance/1 -> Add/1
  Estimated State/1 -> State Feedback Gain/1
  State Feedback Gain/1 -> Add/2
  Add/1 -> Out1/1, Mux/1
  ACE/1 -> Mux/2
  Mux/1 -> Extended-State Observer Controller A3/1

== system DecentralizedLFADRC/LFC with State Feedback/Area 3/G10 Turbine and Generator ==
  u : Inport
  G10 Governor : cstblocks/LTI System  sys=Gg10  IC=[]
  G10 Transient Droop Compensation : cstblocks/LTI System  sys=Gdc10  IC=[]
  G10 Turbine : cstblocks/LTI System  sys=Gt10  IC=[]
  dP_m : Outport  VectorParamsAs1DForOutWhenUnconnected=off
  wires:
  u/1 -> G10 Governor/1
  G10 Transient Droop Compensation/1 -> G10 Turbine/1
  G10 Turbine/1 -> dP_m/1
  G10 Governor/1 -> G10 Transient Droop Compensation/1

== system DecentralizedLFADRC/LFC with State Feedback/Area 3/G8 Turbine and Generator ==
  u : Inport
  G8 Governor : cstblocks/LTI System  sys=Gg8  IC=[]
  G8 Transient Droop Compensation : cstblocks/LTI System  sys=Gdc8  IC=[]
  G8 Turbine : cstblocks/LTI System  sys=Gt8  IC=[]
  dP_m : Outport  VectorParamsAs1DForOutWhenUnconnected=off
  wires:
  u/1 -> G8 Governor/1
  G8 Transient Droop Compensation/1 -> G8 Turbine/1
  G8 Turbine/1 -> dP_m/1
  G8 Governor/1 -> G8 Transient Droop Compensation/1

== system DecentralizedLFADRC/LFC with State Feedback/Area 3/G9 Turbine and Generator ==
  u : Inport
  G9 Governor : cstblocks/LTI System  sys=Gg9  IC=[]
  G9 Turbine : cstblocks/LTI System  sys=Gt9  IC=[]
  dP_m : Outport  VectorParamsAs1DForOutWhenUnconnected=off
  wires:
  G9 Turbine/1 -> dP_m/1
  G9 Governor/1 -> G9 Turbine/1
  u/1 -> G9 Governor/1

== system DecentralizedLFADRC/LFC with State Feedback/Area 3/Load and Interarea Power Flow ==
  P_23 : Inport
  P_31 : Inport  Port=2
  Add : Sum  Inputs=+-
  Add1 : Sum  Inputs=+++
  Gain1 : Gain  Gain=-1
  LTI System : cstblocks/LTI System  sys=tf(100,conv([1 10],[1 10]))  IC=[]
  "Load Disturbance Area 3 " : Subsystem
  PV Negative Load Area 3 : Subsystem
  Random Number : RandomNumber  Mean=75  Variance=10  SampleTime=35
  Rate Transition : RateTransition
  Scope : Scope
  P_load : Outport  VectorParamsAs1DForOutWhenUnconnected=off
  wires:
  "Load Disturbance Area 3 "/1(P_load) -> Gain1/1
  Gain1/1 -> Add1/2
  PV Negative Load Area 3/1(P_pv) -> Add1/3
  P_23/1 -> Add/1
  P_31/1 -> Add/2
  Add/1 -> Add1/1
  Add1/1 -> P_load/1
  LTI System/1 -> Scope/1, PV Negative Load Area 3/1(Irradiance)
  Random Number/1 -> Rate Transition/1
  Rate Transition/1 -> LTI System/1

== system DecentralizedLFADRC/LFC with State Feedback/Area 3/PV Generator 3  ==
  u : Inport
  PV Dynamics for LFC Participation : cstblocks/LTI System  sys=Gpv_LFC  IC=[]
  dP_pv : Outport  VectorParamsAs1DForOutWhenUnconnected=off
  wires:
  PV Dynamics for LFC Participation/1 -> dP_pv/1
  u/1 -> PV Dynamics for LFC Participation/1

== system DecentralizedLFADRC/LFC with State Feedback/Area 3/Wind Turbine 3 ==
  u : Inport
  Blade Characteristic : Gain  Gain=kpc
  First order lag : cstblocks/LTI System  sys=Gwl  IC=[]
  Pitch actuator : cstblocks/LTI System  sys=Gwp  IC=[]
  d_Pw : Outport  VectorParamsAs1DForOutWhenUnconnected=off
  wires:
  Pitch actuator/1 -> First order lag/1
  u/1 -> Pitch actuator/1
  First order lag/1 -> Blade Characteristic/1
  Blade Characteristic/1 -> d_Pw/1

== system DecentralizedLFADRC/LFC with ADRC/Area 1/ADRC Controller A1 ==
  ACE : Inport
  Add : Sum  Inputs=-+
  Estimated State : Gain  Gain=X_hat_1  Multiplication=Matrix(K*u) (u vector)
  Estimated disturbance : Gain  Gain=Xi_hat_1  Multiplication=Matrix(K*u) (u vector)
  Mux : Mux  Inputs=2
  State Feedback Gain : Gain  Gain=K1  Multiplication=Matrix(K*u)
  State-Space : StateSpace  A=A_obs_1  B=B_obs_1  C=C_obs_1  D=D_obs_1  InitialCondition=0
  Out1 : Outport  VectorParamsAs1DForOutWhenUnconnected=off
  wires:
  Mux/1 -> State-Space/1
  ACE/1 -> Mux/2
  Add/1 -> Mux/1, Out1/1
  State Feedback Gain/1 -> Add/2
  Estimated State/1 -> State Feedback Gain/1
  Estimated disturbance/1 -> Add/1
  State-Space/1 -> Estimated State/1, Estimated disturbance/1

== system DecentralizedLFADRC/LFC with ADRC/Area 1/G1 Turbine and Generator ==
  u : Inport
  G1 Governor : cstblocks/LTI System  sys=Gg1  IC=[]
  G1 Turbine : cstblocks/LTI System  sys=Gt1  IC=[]
  dP_m : Outport  VectorParamsAs1DForOutWhenUnconnected=off
  wires:
  u/1 -> G1 Governor/1
  G1 Governor/1 -> G1 Turbine/1
  G1 Turbine/1 -> dP_m/1

== system DecentralizedLFADRC/LFC with ADRC/Area 1/G2 Turbine and Generator ==
  u : Inport
  G2 Governor : cstblocks/LTI System  sys=Gg2  IC=[]
  G2 Transient Droop Compensation : cstblocks/LTI System  sys=Gdc2  IC=[]
  G2 Turbine : cstblocks/LTI System  sys=Gt2  IC=[]
  dP_m : Outport  VectorParamsAs1DForOutWhenUnconnected=off
  wires:
  u/1 -> G2 Governor/1
  G2 Transient Droop Compensation/1 -> G2 Turbine/1
  G2 Turbine/1 -> dP_m/1
  G2 Governor/1 -> G2 Transient Droop Compensation/1

== system DecentralizedLFADRC/LFC with ADRC/Area 1/G3 Turbine and Generator ==
  u : Inport
  G3 Governor : cstblocks/LTI System  sys=Gg3  IC=[]
  G3 Transient Droop Compensation : cstblocks/LTI System  sys=Gdc3  IC=[]
  G3 Turbine : cstblocks/LTI System  sys=Gt3  IC=[]
  dP_m : Outport  VectorParamsAs1DForOutWhenUnconnected=off
  wires:
  u/1 -> G3 Governor/1
  G3 Transient Droop Compensation/1 -> G3 Turbine/1
  G3 Governor/1 -> G3 Transient Droop Compensation/1
  G3 Turbine/1 -> dP_m/1

== system DecentralizedLFADRC/LFC with ADRC/Area 1/Load and Interarea Power Flow ==
  P_12 : Inport
  P_31 : Inport  Port=2
  Add : Sum  Inputs=-+
  Add1 : Sum  Inputs=+++
  Gain1 : Gain  Gain=-1
  LTI System : cstblocks/LTI System  sys=tf(10,conv([1 10],[1 10]))  IC=[]
  "Load Disturbance Area 1 " : Subsystem
  PV Negative Load Area 1 : Subsystem
  Random Number : RandomNumber  Mean=10  Variance=10  SampleTime=5
  Rate Transition : RateTransition
  Scope1 : Scope
  P_load : Outport  VectorParamsAs1DForOutWhenUnconnected=off
  wires:
  Rate Transition/1 -> LTI System/1
  Random Number/1 -> Rate Transition/1
  LTI System/1 -> PV Negative Load Area 1/1(Irradiance)
  Add1/1 -> P_load/1
  Add/1 -> Add1/1
  P_31/1 -> Add/2
  P_12/1 -> Add/1
  PV Negative Load Area 1/1(P_pv) -> Scope1/1, Add1/3
  Gain1/1 -> Add1/2
  "Load Disturbance Area 1 "/1(P_load) -> Gain1/1

== system DecentralizedLFADRC/LFC with ADRC/Area 1/PV Generator 1  ==
  u : Inport
  PV Dynamics for LFC Participation : cstblocks/LTI System  sys=Gpv_LFC  IC=[]
  dP_pv : Outport  VectorParamsAs1DForOutWhenUnconnected=off
  wires:
  u/1 -> PV Dynamics for LFC Participation/1
  PV Dynamics for LFC Participation/1 -> dP_pv/1

== system DecentralizedLFADRC/LFC with ADRC/Area 1/Wind Turbine 1 ==
  u : Inport
  Blade Characteristic : Gain  Gain=kpc
  First order lag : cstblocks/LTI System  sys=Gwl  IC=[]
  Pitch actuator : cstblocks/LTI System  sys=Gwp  IC=[]
  d_Pw : Outport  VectorParamsAs1DForOutWhenUnconnected=off
  wires:
  Blade Characteristic/1 -> d_Pw/1
  First order lag/1 -> Blade Characteristic/1
  u/1 -> Pitch actuator/1
  Pitch actuator/1 -> First order lag/1

== system DecentralizedLFADRC/LFC with ADRC/Area 2/ADRC Controller A2 ==
  ACE : Inport
  Add : Sum  Inputs=-+
  Estimated State : Gain  Gain=X_hat_2  Multiplication=Matrix(K*u) (u vector)
  Estimated disturbance : Gain  Gain=Xi_hat_2  Multiplication=Matrix(K*u) (u vector)
  Extended-State Observer Controller A2 : StateSpace  A=A_obs_2  B=B_obs_2  C=C_obs_2  D=D_obs_2  InitialCondition=0
  Mux : Mux  Inputs=2
  State Feedback Gain : Gain  Gain=K2  Multiplication=Matrix(K*u)
  Out1 : Outport  VectorParamsAs1DForOutWhenUnconnected=off
  wires:
  Mux/1 -> Extended-State Observer Controller A2/1
  ACE/1 -> Mux/2
  Add/1 -> Mux/1, Out1/1
  State Feedback Gain/1 -> Add/2
  Estimated State/1 -> State Feedback Gain/1
  Estimated disturbance/1 -> Add/1
  Extended-State Observer Controller A2/1 -> Estimated State/1, Estimated disturbance/1

== system DecentralizedLFADRC/LFC with ADRC/Area 2/G4 Turbine and Generator ==
  u : Inport
  G4 Governor : cstblocks/LTI System  sys=Gg4  IC=[]
  G4 Turbine : cstblocks/LTI System  sys=Gt4  IC=[]
  dP_m : Outport  VectorParamsAs1DForOutWhenUnconnected=off
  wires:
  u/1 -> G4 Governor/1
  G4 Governor/1 -> G4 Turbine/1
  G4 Turbine/1 -> dP_m/1

== system DecentralizedLFADRC/LFC with ADRC/Area 2/G5 Turbine and Generator ==
  u : Inport
  G5 Governor : cstblocks/LTI System  sys=Gg5  IC=[]
  G5 Transient Droop Compensation : cstblocks/LTI System  sys=Gdc5  IC=[]
  G5 Turbine : cstblocks/LTI System  sys=Gt5  IC=[]
  dP_m : Outport  VectorParamsAs1DForOutWhenUnconnected=off
  wires:
  G5 Governor/1 -> G5 Transient Droop Compensation/1
  G5 Turbine/1 -> dP_m/1
  G5 Transient Droop Compensation/1 -> G5 Turbine/1
  u/1 -> G5 Governor/1

== system DecentralizedLFADRC/LFC with ADRC/Area 2/G6 Turbine and Generator ==
  u : Inport
  G6 Governor : cstblocks/LTI System  sys=Gg6  IC=[]
  G6 Transient Droop Compensation : cstblocks/LTI System  sys=Gdc6  IC=[]
  G6 Turbine : cstblocks/LTI System  sys=Gt6  IC=[]
  dP_m : Outport  VectorParamsAs1DForOutWhenUnconnected=off
  wires:
  G6 Governor/1 -> G6 Transient Droop Compensation/1
  G6 Turbine/1 -> dP_m/1
  G6 Transient Droop Compensation/1 -> G6 Turbine/1
  u/1 -> G6 Governor/1

== system DecentralizedLFADRC/LFC with ADRC/Area 2/G7 Turbine and Generator ==
  u : Inport
  G7 Governor : cstblocks/LTI System  sys=Gg7  IC=[]
  G7 Transient Droop Compensation : cstblocks/LTI System  sys=Gdc7  IC=[]
  G7 Turbine : cstblocks/LTI System  sys=Gt7  IC=[]
  dP_m : Outport  VectorParamsAs1DForOutWhenUnconnected=off
  wires:
  u/1 -> G7 Governor/1
  G7 Transient Droop Compensation/1 -> G7 Turbine/1
  G7 Turbine/1 -> dP_m/1
  G7 Governor/1 -> G7 Transient Droop Compensation/1

== system DecentralizedLFADRC/LFC with ADRC/Area 2/Load and Interarea Power Flow ==
  P_12 : Inport
  P_23 : Inport  Port=2
  Add : Sum  Inputs=+-
  Add1 : Sum  Inputs=+++
  Gain1 : Gain  Gain=-1
  LTI System : cstblocks/LTI System  sys=tf(10,conv([1 10],[1 10]))  IC=[]
  "Load Disturbance Area 2 " : Subsystem
  PV Negative Load Area 2 : Subsystem
  Random Number : RandomNumber  Mean=15  Variance=15  SampleTime=10
  Rate Transition : RateTransition
  Scope : Scope
  P_load : Outport  VectorParamsAs1DForOutWhenUnconnected=off
  wires:
  Rate Transition/1 -> LTI System/1
  Random Number/1 -> Rate Transition/1
  LTI System/1 -> PV Negative Load Area 2/1(Irradiance), Scope/1
  Add1/1 -> P_load/1
  Add/1 -> Add1/1
  P_23/1 -> Add/2
  P_12/1 -> Add/1
  PV Negative Load Area 2/1(P_pv) -> Add1/3
  Gain1/1 -> Add1/2
  "Load Disturbance Area 2 "/1(P_load) -> Gain1/1

== system DecentralizedLFADRC/LFC with ADRC/Area 2/PV Generator 2  ==
  u : Inport
  PV Dynamics for LFC Participation : cstblocks/LTI System  sys=Gpv_LFC  IC=[]
  dP_pv : Outport  VectorParamsAs1DForOutWhenUnconnected=off
  wires:
  u/1 -> PV Dynamics for LFC Participation/1
  PV Dynamics for LFC Participation/1 -> dP_pv/1

== system DecentralizedLFADRC/LFC with ADRC/Area 3/ADRC Controller A3 ==
  ACE : Inport
  Add : Sum  Inputs=-+
  Estimated State : Gain  Gain=X_hat_3  Multiplication=Matrix(K*u) (u vector)
  Estimated disturbance : Gain  Gain=Xi_hat_3  Multiplication=Matrix(K*u) (u vector)
  Extended-State Observer Controller A3 : StateSpace  A=A_obs_3  B=B_obs_3  C=C_obs_3  D=D_obs_3  InitialCondition=0
  Mux : Mux  Inputs=2
  State Feedback Gain : Gain  Gain=K3  Multiplication=Matrix(K*u)
  Out1 : Outport  VectorParamsAs1DForOutWhenUnconnected=off
  wires:
  Mux/1 -> Extended-State Observer Controller A3/1
  ACE/1 -> Mux/2
  Add/1 -> Mux/1, Out1/1
  State Feedback Gain/1 -> Add/2
  Estimated State/1 -> State Feedback Gain/1
  Estimated disturbance/1 -> Add/1
  Extended-State Observer Controller A3/1 -> Estimated State/1, Estimated disturbance/1

== system DecentralizedLFADRC/LFC with ADRC/Area 3/G10 Turbine and Generator ==
  u : Inport
  G10 Governor : cstblocks/LTI System  sys=Gg10  IC=[]
  G10 Transient Droop Compensation : cstblocks/LTI System  sys=Gdc10  IC=[]
  G10 Turbine : cstblocks/LTI System  sys=Gt10  IC=[]
  dP_m : Outport  VectorParamsAs1DForOutWhenUnconnected=off
  wires:
  G10 Governor/1 -> G10 Transient Droop Compensation/1
  G10 Turbine/1 -> dP_m/1
  G10 Transient Droop Compensation/1 -> G10 Turbine/1
  u/1 -> G10 Governor/1

== system DecentralizedLFADRC/LFC with ADRC/Area 3/G8 Turbine and Generator ==
  u : Inport
  G8 Governor : cstblocks/LTI System  sys=Gg8  IC=[]
  G8 Transient Droop Compensation : cstblocks/LTI System  sys=Gdc8  IC=[]
  G8 Turbine : cstblocks/LTI System  sys=Gt8  IC=[]
  dP_m : Outport  VectorParamsAs1DForOutWhenUnconnected=off
  wires:
  G8 Governor/1 -> G8 Transient Droop Compensation/1
  G8 Turbine/1 -> dP_m/1
  G8 Transient Droop Compensation/1 -> G8 Turbine/1
  u/1 -> G8 Governor/1

== system DecentralizedLFADRC/LFC with ADRC/Area 3/G9 Turbine and Generator ==
  u : Inport
  G9 Governor : cstblocks/LTI System  sys=Gg9  IC=[]
  G9 Turbine : cstblocks/LTI System  sys=Gt9  IC=[]
  dP_m : Outport  VectorParamsAs1DForOutWhenUnconnected=off
  wires:
  u/1 -> G9 Governor/1
  G9 Governor/1 -> G9 Turbine/1
  G9 Turbine/1 -> dP_m/1

== system DecentralizedLFADRC/LFC with ADRC/Area 3/Load and Interarea Power Flow ==
  P_23 : Inport
  P_31 : Inport  Port=2
  Add : Sum  Inputs=+-
  Add1 : Sum  Inputs=+++
  Gain1 : Gain  Gain=-1
  LTI System : cstblocks/LTI System  sys=tf(100,conv([1 10],[1 10]))  IC=[]
  "Load Disturbance Area 3 " : Subsystem
  PV Negative Load Area 3 : Subsystem
  Random Number : RandomNumber  Mean=75  Variance=10  SampleTime=35
  Rate Transition : RateTransition
  Scope : Scope
  P_load : Outport  VectorParamsAs1DForOutWhenUnconnected=off
  wires:
  Rate Transition/1 -> LTI System/1
  Random Number/1 -> Rate Transition/1
  LTI System/1 -> PV Negative Load Area 3/1(Irradiance), Scope/1
  Add1/1 -> P_load/1
  Add/1 -> Add1/1
  P_31/1 -> Add/2
  P_23/1 -> Add/1
  PV Negative Load Area 3/1(P_pv) -> Add1/3
  Gain1/1 -> Add1/2
  "Load Disturbance Area 3 "/1(P_load) -> Gain1/1

== system DecentralizedLFADRC/LFC with ADRC/Area 3/PV Generator 3  ==
  u : Inport
  PV Dynamics for LFC Participation : cstblocks/LTI System  sys=Gpv_LFC  IC=[]
  dP_pv : Outport  VectorParamsAs1DForOutWhenUnconnected=off
  wires:
  u/1 -> PV Dynamics for LFC Participation/1
  PV Dynamics for LFC Participation/1 -> dP_pv/1

== system DecentralizedLFADRC/LFC with ADRC/Area 3/Wind Turbine 3 ==
  u : Inport
  Blade Characteristic : Gain  Gain=kpc
  First order lag : cstblocks/LTI System  sys=Gwl  IC=[]
  Pitch actuator : cstblocks/LTI System  sys=Gwp  IC=[]
  d_Pw : Outport  VectorParamsAs1DForOutWhenUnconnected=off
  wires:
  Blade Characteristic/1 -> d_Pw/1
  First order lag/1 -> Blade Characteristic/1
  u/1 -> Pitch actuator/1
  Pitch actuator/1 -> First order lag/1
